simulink model "V2ModelWs"  (R2018b)
settings: Solver=ode45  StartTime=0.0  StopTime=20.0  MaxStep=0.1  RelTol=1e-3  EnableMultiTasking=on
model workspace (MAT data in the model file):
  c1 = 1
  c2 = 1
  c3 = 1
  c4 = 1
  m1 = 2
  m2 = 2
  m3 = 2
  v1 = 0
  v2 = 0
  v3 = 0
  x1 = -1.5
  x2 = 0
  x3 = 1
settings Model: Creator=Reichl  LastModifiedBy=Reichl
settings DataIOCC: SaveFormat=Array  SignalLoggingSaveFormat=ModelDataLogs
settings OptimizationCC: ExpressionDepthLimit=2147483647  LifeSpan=inf
settings DebuggingCC: UnderspecifiedInitializationDetection=Classic  MergeDetectMultiDrivingBlocksExec=none  SolverPrmCheckMsg=warning  FcnCallInpInsideContextMsg=warning  AllowSymbolicDim=off  StateNameClashWarn=warning  SFUnexpectedBacktrackingDiag=warning  SFNoUnconditionalDefaultTransitionDiag=warning  SFExecutionAtInitializationDiag=none
settings HardwareCC: ProdBitPerPointer=32  ProdBitPerSizeT=32  ProdBitPerPtrDiffT=32  ProdLargestAtomicFloat=None  ProdIntDivRoundTo=Undefined  ProdEndianess=Unspecified  ProdWordSize=32  ProdHWDeviceType=32-bit Generic
settings ModelReferenceCC: PropagateSignalLabelsOutOfModel=off
settings SFSimCC: SimUseLocalCustomCode=off
settings RTWCC: RTWUseLocalCustomCode=off
settings CodeAppCC: StateflowObjectComments=on
settings GRTTargetCC: TargetLangStandard=C89/C90 (ANSI)  GeneratePreprocessorConditionals=Disable all  CombineOutputUpdateFcns=off  GRTInterface=on
settings ConfigComp: CovMetricSettings=dw  CovHtmlReporting=on  CovSaveCumulativeToWorkspaceVar=on  CovSaveSingleToWorkspaceVar=on  CovExternalEMLEnable=off  CovSFcnEnable=off

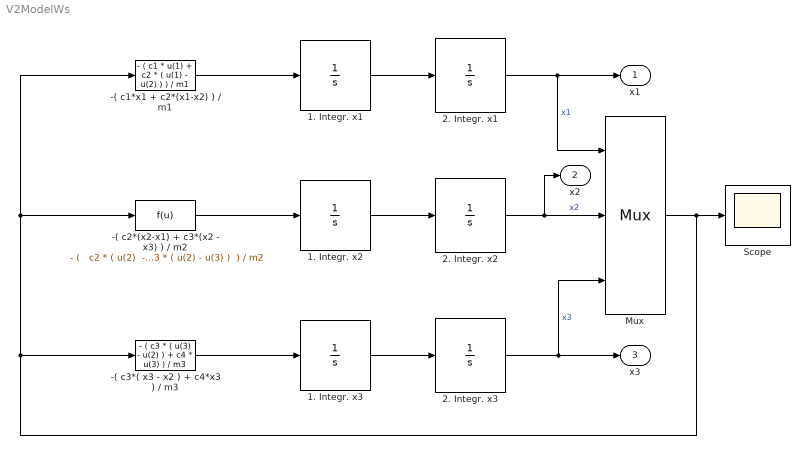
== system V2ModelWs ==
  -( c1*x1 + c2*(x1-x2) ) / m1 : Fcn  Expr="- (   c1 * u(1)  +  c2 * ( u(1) - u(2) )  ) / m1"
  -( c2*(x2-x1) + c3*(x2 - x3) ) / m2 : Fcn  Expr="- (   c2 * ( u(2)  -u(1) )  +  c3 * ( u(2) - u(3) )  ) / m2"
  -( c3*( x3 - x2 ) + c4*x3 ) / m3 : Fcn  Expr="- (  c3 * ( u(3) - u(2) )  +  c4 * u(3)  ) / m3"
  1. Integr. x1 : Integrator  InitialCondition=v1
  1. Integr. x2 : Integrator  InitialCondition=v2
  1. Integr. x3 : Integrator  InitialCondition=v3
  2. Integr. x1 : Integrator  InitialCondition=x1
  2. Integr. x2 : Integrator  InitialCondition=x2
  2. Integr. x3 : Integrator  InitialCondition=x3
  Mux : Mux  Inputs=3
      settings: DisplayOption=signals
  Scope : Scope
  x1 : Outport
  x2 : Outport  Port=2
  x3 : Outport  Port=3
  wires:
  1. Integr. x1/1 -> 2. Integr. x1/1
  1. Integr. x2/1 -> 2. Integr. x2/1
  1. Integr. x3/1 -> 2. Integr. x3/1
  Mux/1 -> Scope/1, -( c3*( x3 - x2 ) + c4*x3 ) / m3/1, -( c1*x1 + c2*(x1-x2) ) / m1/1, -( c2*(x2-x1) + c3*(x2 - x3) ) / m2/1
  2. Integr. x2/1 -> x2/1, Mux/2  "x2"
  2. Integr. x1/1 -> Mux/1, x1/1  "x1"
  2. Integr. x3/1 -> x3/1, Mux/3  "x3"
  -( c1*x1 + c2*(x1-x2) ) / m1/1 -> 1. Integr. x1/1
  -( c2*(x2-x1) + c3*(x2 - x3) ) / m2/1 -> 1. Integr. x2/1
  -( c3*( x3 - x2 ) + c4*x3 ) / m3/1 -> 1. Integr. x3/1
